simulink model "Three_Phase_Inverter"  (R2020a)
settings: Solver=VariableStepAuto  StartTime=0.0  StopTime=10.0  RelTol=1e-3
libraries: powerlib x15
settings Model: Creator=Kritika  LastModifiedBy=Kritika

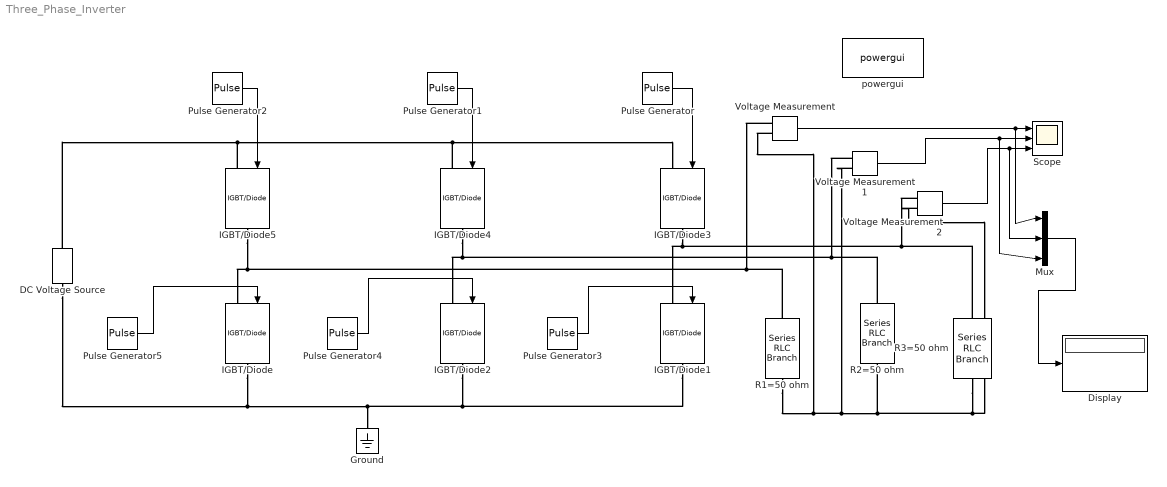
== system Three_Phase_Inverter ==
  DC Voltage Source : powerlib/Electrical Sources/DC Voltage Source  Amplitude=200  Measurements=None
  Display : Display
      settings: Decimation=200
  Ground : powerlib/Elements/Ground  LConnTagsString=a
  IGBT/Diode{,1..5} (6 alike) : powerlib/Power Electronics/IGBT//Diode  Ron=1e-3  Rs=1e5  Cs=inf  Measurements=off
  Mux : Mux  Inputs=3
  Pulse Generator : DiscretePulseGenerator  PulseType=Time based  Period=2e-3  PulseWidth=50  PhaseDelay=(2e-3)*(4/6)
  Pulse Generator1 : DiscretePulseGenerator  PulseType=Time based  Period=2e-3  PulseWidth=50  PhaseDelay=(2e-3)*(2/6)
  Pulse Generator2 : DiscretePulseGenerator  PulseType=Time based  Period=2e-3  PulseWidth=50
  Pulse Generator3 : DiscretePulseGenerator  PulseType=Time based  Period=2e-3  PulseWidth=50  PhaseDelay=(2e-3)*(1/6)
  Pulse Generator4 : DiscretePulseGenerator  PulseType=Time based  Period=2e-3  PulseWidth=50  PhaseDelay=(2e-3)*(5/6)
  Pulse Generator5 : DiscretePulseGenerator  PulseType=Time based  Period=2e-3  PulseWidth=50  PhaseDelay=(2e-3)*(3/6)
  R1=50 ohm : powerlib/Elements/Series RLC Branch  LConnTagsString=__new0  RConnTagsString=__new0  BranchType=R  Resistance=50  Inductance=1e-3  SetiL0=off  InitialCurrent=0  Capacitance=1e-6  Setx0=off  InitialVoltage=0  Measurements=None
  R2=50 ohm : powerlib/Elements/Series RLC Branch  LConnTagsString=__new0  RConnTagsString=__new0  BranchType=R  Resistance=50  Inductance=1e-3  SetiL0=off  InitialCurrent=0  Capacitance=1e-6  Setx0=off  InitialVoltage=0  Measurements=None
  R3=50 ohm : powerlib/Elements/Series RLC Branch  LConnTagsString=__new0  RConnTagsString=__new0  BranchType=R  Resistance=50  Inductance=1e-3  SetiL0=off  InitialCurrent=0  Capacitance=1e-6  Setx0=off  InitialVoltage=0  Measurements=None
  Scope : Scope  NumInputPorts=3
  Voltage Measurement : powerlib/Measurements/Voltage Measurement  PhasorSimulation=off  OutputType=Complex  PSBequivalent=0
  Voltage Measurement1 : powerlib/Measurements/Voltage Measurement  PhasorSimulation=off  OutputType=Complex  PSBequivalent=0
  Voltage Measurement2 : powerlib/Measurements/Voltage Measurement  PhasorSimulation=off  OutputType=Complex  PSBequivalent=0
  powergui : powerlib/powergui  Priority=1  SimulationMode=Continuous  SampleTime=50e-6  frequency=60  Iterations=50  frequencyindice=0  Pbase=100e6  ErrMax=1e-4  UnitsV=kV  UnitsW=MW  buscounter=0  FunctionMessages=off  echomessages=off  EnableUseOfTLC=off  CurrentSourceSwitches=off  DisableSnubberDevices=off  DisableRonSwitches=off  DisableVfSwitches=off  DisplayEquations=off  AutomaticDiscreteSolvers=off  SolverType=Tustin/Backward Euler (TBE)  Interpol=off  ExternalGateDelay=off  methode=off  Ts=100  x0status=blocks  SPID=on  SwTol=0  HookPort=off  NonlinearTolerance=1e-4  nMaxIteration=100  ContinueOnMaxIteration=off  RestoreLinks=warning  ResistiveCurrentMeasurement=off  Frange=[0:2:500]  Ylog=off  Xlog=on  ShowGrid=off  save=off  variable=ZData  structure=0  ZoomFFT=off  StartTime=0.0  cycles=1  DisplayStyle=1  fundamental=60  FreqAxis=off  MaxFrequency=1000  frequencyindicesteady=1  RmsSteady=1  display=off
  wires:
  Pulse Generator2/1 -> IGBT/Diode5/1
  Pulse Generator1/1 -> IGBT/Diode4/1
  Pulse Generator/1 -> IGBT/Diode3/1
  Pulse Generator4/1 -> IGBT/Diode2/1
  Pulse Generator3/1 -> IGBT/Diode1/1
  Pulse Generator5/1 -> IGBT/Diode/1
  Voltage Measurement2/1 -> Mux/2, Scope/3
  Voltage Measurement1/1 -> Mux/3, Scope/2
  Voltage Measurement/1 -> Mux/1, Scope/1
  Mux/1 -> Display/1
  connections:
  DC Voltage Source/LConn1 -- IGBT/Diode/RConn1 -- IGBT/Diode1/RConn1 -- IGBT/Diode2/RConn1 -- Ground/LConn1
  DC Voltage Source/RConn1 -- IGBT/Diode5/LConn1 -- IGBT/Diode4/LConn1 -- IGBT/Diode3/LConn1
  IGBT/Diode5/RConn1 -- IGBT/Diode/LConn1 -- R1=50 ohm/LConn1 -- Voltage Measurement/LConn1
  IGBT/Diode4/RConn1 -- IGBT/Diode2/LConn1 -- R2=50 ohm/LConn1 -- Voltage Measurement1/LConn1
  IGBT/Diode3/RConn1 -- IGBT/Diode1/LConn1 -- R3=50 ohm/LConn1 -- Voltage Measurement2/LConn1
  R1=50 ohm/RConn1 -- Voltage Measurement1/LConn2 -- Voltage Measurement2/LConn2 -- R3=50 ohm/RConn1 -- R2=50 ohm/RConn1 -- Voltage Measurement/LConn2
